simulink library "Max_Run_Time"  (Simulink 8.2)
settings: Solver=ode45  StartTime=0.0  StopTime=10.0  RelTol=1e-3
libraries: simulink x1
settings Model: Creator=lena.frank  LastModifiedBy=drhf

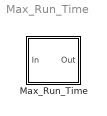
== system Max_Run_Time ==
  Max_Run_Time : Subsystem  mask(Maximum Running Time){tmaxrun=5}
      mask prompts: tmaxrun "Maximum operation time in s"
      mask help: Keeps the output to the input level until either the maximum running time is reached or the input is set to zero.
      mask Help: web(fullfile(path_carnot('help'),'Max_Run_Time.html'),'-helpbrowser')
      mask Display:
      | plot(-20,-30,120,100,[10,20,40,60,80,90,90,80,60,40,20,10,10],[40,20,10,10,20,40,60,80,90,90,80,60,40],[55,46],[95,95],[50,50],[90,95],[50,50,24],[88,50,66],[10,13],[50,50],[90,87],[50,50],[50,50],[10,15])
      | disp('\n\nMax On')

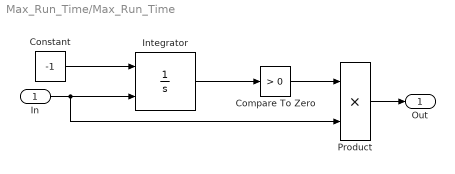
== system Max_Run_Time/Max_Run_Time ==
  In : Inport
  Compare To Zero : simulink/Logic and Bit Operations/Compare To Zero  relop=>  OutDataTypeStr=uint8
  Constant : Constant  Value=-1
  Integrator : Integrator  ExternalReset=rising  InitialCondition=tmaxrun  LimitOutput=on  LowerSaturationLimit=0
  Product : Product  RndMeth=Zero
  Out : Outport
  wires:
  Product/1 -> Out/1
  In/1 -> Integrator/2, Product/2
  Compare To Zero/1 -> Product/1
  Integrator/1 -> Compare To Zero/1
  Constant/1 -> Integrator/1
